simulink model "TVModel_Simulation_21"  (R2021b)
settings: Solver=FixedStepDiscrete  StartTime=0.0  StopTime=250  FixedStep=0.02  MaxStep=0.01  RelTol=1e-3
undefined symbols (not defined in the file or in its folder): MB, TV, TV_OLD
libraries: simulink x22, simulink_extras x14, eeGeneralControl x13, slpidlib x8, fuzblock x4, controlLib x4, cstblocks x3, dspstat3 x2, eeSlidingModeController x1, sharedTrackingLibrary x1
(part 3 of 9)

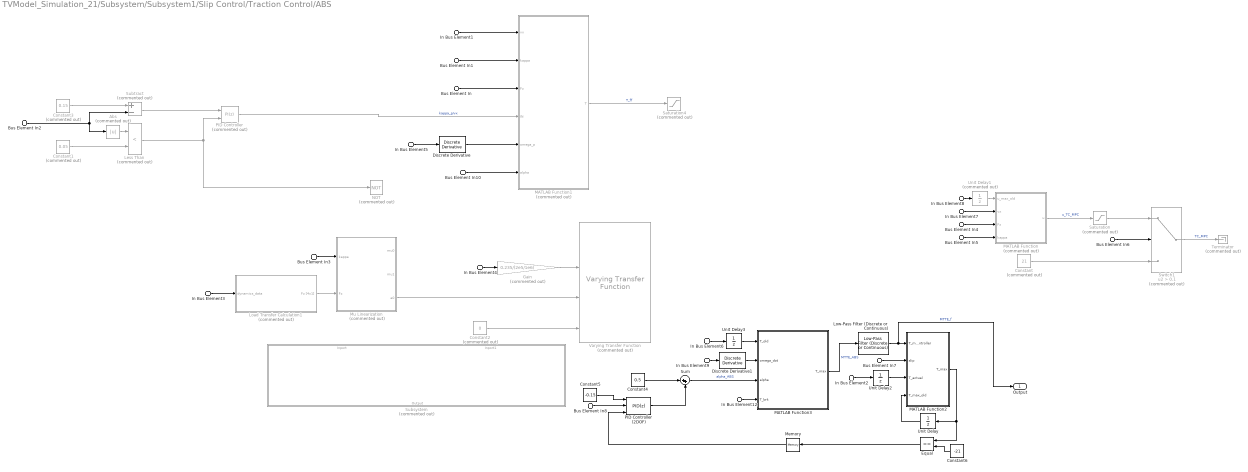
== system TVModel_Simulation_21/Subsystem/Subsystem1/Slip Control/Traction Control/ABS ==
  In Bus Element3 : Inport  PortName=dynamics_data
  In Bus Element1 : Inport  PortName=dynamics_data  Element=vx
  In Bus Element4 : Inport  PortName=dynamics_data  Element=vx
  In Bus Element7 : Inport  PortName=dynamics_data  Element=vx
  In Bus Element5 : Inport  PortName=dynamics_data  Element=omega_wheels
  In Bus Element9 : Inport  PortName=dynamics_data  Element=omega_wheels
  In Bus Element12 : Inport  PortName=dynamics_data  Element=brake_torque
  Bus Element In{1..3,5..8} (7 alike) : Inport  Port=2  PortName=slip_ratio
  Bus Element In10 : Inport  Port=3  PortName=slip_angles
  Bus Element In : Inport  Port=4  PortName=Fz
  Bus Element In4 : Inport  Port=4  PortName=Fz
  In Bus Element8 : Inport  Port=5  PortName=tv
  In Bus Element2 : Inport  Port=5  PortName=tv
  In Bus Element6 : Inport  Port=5  PortName=tv
  Abs : Abs  Commented=on
  Constant : Constant  Commented=on  Value=21
  Constant1 : Constant  Commented=on  Value=0.05
  Constant2 : Constant  Commented=on  Value=0
  Constant3 : Constant  Commented=on  Value=0.15
  Constant4 : Constant  Value=0.5
  Constant5 : Constant  Value=-0.15
  Constant6 : Constant  Value=-21
  Discrete Derivative : simulink/Discrete/Discrete Derivative  gainval=1.0  ICPrevScaledInput=0.0  OutMin=[]  OutMax=[]  OutDataType=fixdt(1, 16)  OutScaling=2^-10  DoSatur=off
  Discrete Derivative1 : simulink/Discrete/Discrete Derivative  gainval=1.0  ICPrevScaledInput=0.0  OutMin=[]  OutMax=[]  OutDataType=fixdt(1, 16)  OutScaling=2^-10  DoSatur=off
  Equal : RelationalOperator  Operator===  OutDataTypeStr=boolean  RndMeth=Simplest
  Gain : Gain  Commented=on  Gain=0.235/(2e5/1e6)
  Less Than : RelationalOperator  Commented=on  Operator=<  OutDataTypeStr=boolean  RndMeth=Simplest
  Load Transfer Calculation1 : Subsystem  Commented=on
  Low-Pass Filter (Discrete or Continuous) : eeGeneralControl/Low-Pass Filter (Discrete or Continuous)  K=1  T=0.1  B=inf  A=-inf  init_option=Inherited from block input  x0=0  Ts=-1
  MATLAB Function : MATLAB Function  Commented=on  TreatAsAtomicUnit=on
  MATLAB Function1 : MATLAB Function  Commented=on  TreatAsAtomicUnit=on
  MATLAB Function2 : MATLAB Function  TreatAsAtomicUnit=on
  MATLAB Function3 : MATLAB Function  TreatAsAtomicUnit=on
  Memory : Memory  InitialCondition=1  InheritSampleTime=on
  Mu Linearization : MATLAB Function  Commented=on  TreatAsAtomicUnit=on
  NOT : Logic  Commented=on  Operator=NOT  IconShape=distinctive  AllPortsSameDT=off  OutDataTypeStr=boolean
  PID Controller : slpidlib/PID Controller  Commented=on  Controller=PI  Form=Parallel  TimeDomain=Discrete-time  UseExternalTs=off  SampleTime=-1  IntegratorMethod=Forward Euler  FilterMethod=Forward Euler  ControllerParametersSource=internal  P=0  I=5  D=0  UseFilter=on  N=100  TunerSelectOption=Transfer Function Based (PID Tuner App)  InitialConditionSource=internal  InitialConditionForIntegrator=0  InitialConditionForFilter=0  DifferentiatorICPrevScaledInput=0  ExternalReset=level  TrackingMode=off  Kt=1  LimitOutput=off  SatLimitsSource=internal  UpperSaturationLimit=0  LowerSaturationLimit=-20  LinearizeAsGain=on  AntiWindupMode=clamping  Kb=1  POutMin=[]  POutMax=[]  IOutMin=[]  IOutMax=[]  DOutMin=[]  DOutMax=[]  NOutMin=[]  NOutMax=[]  SumOutMin=[]  SumOutMax=[]  SaturationOutMin=[]  SaturationOutMax=[]  PParamMin=[]  PParamMax=[]  IParamMin=[]  IParamMax=[]  DParamMin=[]  DParamMax=[]  NParamMin=[]  NParamMax=[]  KbParamMin=[]  KbParamMax=[]  KtParamMin=[]  KtParamMax=[]  KbOutMin=[]  KbOutMax=[]  KtOutMin=[]  KtOutMax=[]  IntegratorOutMin=[]  IntegratorOutMax=[]  FilterOutMin=[]  FilterOutMax=[]  SumI1OutMin=[]  SumI1OutMax=[]  SumI2OutMin=[]  SumI2OutMax=[]  SumI3OutMin=[]  SumI3OutMax=[]  SumI4OutMin=[]  SumI4OutMax=[]  SumDOutMin=[]  SumDOutMax=[]  DifferentiatorOutMin=[]  DifferentiatorOutMax=[]  FilterDiffOutCoefMin=[]  FilterDiffOutCoefMax=[]  ReciprocalOutMin=[]  ReciprocalOutMax=[]  SumDenOutMin=[]  SumDenOutMax=[]  SumNumOutMin=[]  SumNumOutMax=[]  DivideOutMin=[]  DivideOutMax=[]  UdiffTsProdOutMin=[]  UdiffTsProdOutMax=[]  NTsProdOutMin=[]  NTsProdOutMax=[]  UintegralTsProdOutMin=[]  UintegralTsProdOutMax=[]  UngainTsProdOutMin=[]  UngainTsProdOutMax=[]  IntegratorContinuousStateAttributes=''  IntegratorStateMustResolveToSignalObject=off  IntegratorRTWStateStorageClass=Auto  FilterContinuousStateAttributes=''  FilterStateMustResolveToSignalObject=off  FilterRTWStateStorageClass=Auto  ParallelPVariant=InternalParameters  IdealPVariant=Disabled  IVariant=InternalParameters  DVariant=Disabled  IntegratorVariant=Discrete  SatVariant=Disabled  AWVariant=Passthrough  PCopyVariant=Disabled  TRVariant=Disabled  FdbkBlocksVariant=Forward  IdealPFdbkVariant=Disabled  SatFdbkVariant=Disabled  DerivativeFilterVariant=Disabled  NVariant=Disabled  NCopyVariant=Disabled_SignalSpec  FilterICVariant=Disabled  IntegratorICVariant=InternalICs  ExternalResetVariant=ExternalReset  TRSumVariant=Passthrough  SumFdbkVariant=Disabled  SumVariant=Sum_PI  TsampFilterVariant=InternalTs  TsampNgainVariant=Passthrough  TsampIntegralVariant=Passthrough  ExternalSaturationOutDataTypeStr=Inherit: Same as second input
  PID Controller (2DOF) : slpidlib/PID Controller (2DOF)  Controller=PID  Form=Parallel  TimeDomain=Discrete-time  UseExternalTs=off  SampleTime=0.02  IntegratorMethod=Forward Euler  FilterMethod=Forward Euler  ControllerParametersSource=internal  P=1  I=1  D=0  UseFilter=on  N=100  b=1  c=1  TunerSelectOption=Transfer Function Based (PID Tuner App)  InitialConditionSource=internal  InitialConditionForIntegrator=0  InitialConditionForFilter=0  DifferentiatorICPrevScaledInput=0  ExternalReset=level  TrackingMode=off  Kt=1  LimitOutput=on  SatLimitsSource=internal  UpperSaturationLimit=2  LowerSaturationLimit=0  LinearizeAsGain=on  AntiWindupMode=clamping  Kb=1  POutMin=[]  POutMax=[]  IOutMin=[]  IOutMax=[]  DOutMin=[]  DOutMax=[]  NOutMin=[]  NOutMax=[]  bOutMin=[]  bOutMax=[]  cOutMin=[]  cOutMax=[]  SumOutMin=[]  SumOutMax=[]  SaturationOutMin=[]  SaturationOutMax=[]  PParamMin=[]  PParamMax=[]  IParamMin=[]  IParamMax=[]  DParamMin=[]  DParamMax=[]  NParamMin=[]  NParamMax=[]  bParamMin=[]  bParamMax=[]  cParamMin=[]  cParamMax=[]  KbParamMin=[]  KbParamMax=[]  KtParamMin=[]  KtParamMax=[]  KbOutMin=[]  KbOutMax=[]  KtOutMin=[]  KtOutMax=[]  IntegratorOutMin=[]  IntegratorOutMax=[]  FilterOutMin=[]  FilterOutMax=[]  SumI1OutMin=[]  SumI1OutMax=[]  SumI2OutMin=[]  SumI2OutMax=[]  SumI3OutMin=[]  SumI3OutMax=[]  SumI4OutMin=[]  SumI4OutMax=[]  SumDOutMin=[]  SumDOutMax=[]  Sum1OutMin=[]  Sum1OutMax=[]  Sum2OutMin=[]  Sum2OutMax=[]  Sum3OutMin=[]  Sum3OutMax=[]  DifferentiatorOutMin=[]  DifferentiatorOutMax=[]  FilterDiffOutCoefMin=[]  FilterDiffOutCoefMax=[]  ReciprocalOutMin=[]  ReciprocalOutMax=[]  SumDenOutMin=[]  SumDenOutMax=[]  SumNumOutMin=[]  SumNumOutMax=[]  DivideOutMin=[]  DivideOutMax=[]  UdiffTsProdOutMin=[]  UdiffTsProdOutMax=[]  NTsProdOutMin=[]  NTsProdOutMax=[]  UintegralTsProdOutMin=[]  UintegralTsProdOutMax=[]  UngainTsProdOutMin=[]  UngainTsProdOutMax=[]  IntegratorContinuousStateAttributes=''  IntegratorStateMustResolveToSignalObject=off  IntegratorRTWStateStorageClass=Auto  FilterContinuousStateAttributes=''  FilterStateMustResolveToSignalObject=off  FilterRTWStateStorageClass=Auto  ParallelPVariant=InternalParameters  IdealPVariant=Disabled  IVariant=InternalParameters  DVariant=InternalParameters  bVariant=InternalParameters  cVariant=InternalParameters  IntegratorVariant=Discrete  SatVariant=Enabled  AWVariant=DiscClampingParallel  PCopyVariant=Disabled  TRVariant=Disabled  FdbkBlocksVariant=Forward  IdealPFdbkVariant=Disabled  SatFdbkVariant=Disabled  DerivativeFilterVariant=ForwardEulerFilter  NVariant=InternalParameters  NCopyVariant=Disabled  FilterICVariant=InternalICsFilter  IntegratorICVariant=InternalICs  ExternalResetVariant=ExternalReset  TRSumVariant=Passthrough  SumFdbkVariant=Disabled  SumVariant=Sum_PID  TsampFilterVariant=InternalTs  TsampNgainVariant=Passthrough  TsampIntegralVariant=Passthrough  ExternalSaturationOutDataTypeStr=Inherit: Same as second input
      settings: SourceProductBaseCode=SL
  Saturation : Saturate  Commented=on  UpperLimit=21  LowerLimit=0
  Saturation4 : Saturate  Commented=on  UpperLimit=21  LowerLimit=2
  Subsystem : Subsystem  Commented=on
  Subtract : Sum  Commented=on  Inputs=+-
  Sum : Sum  Inputs=|++
  Switch1 : Switch  Commented=on  Criteria=u2 > Threshold  Threshold=0.1
  Terminator : Terminator  Commented=on
  Unit Delay : UnitDelay  SampleTime=-1  HasFrameUpgradeWarning=on
  Unit Delay1 : UnitDelay  Commented=on  SampleTime=-1  HasFrameUpgradeWarning=on
  Unit Delay2 : UnitDelay  SampleTime=-1  HasFrameUpgradeWarning=on
  Unit Delay3 : UnitDelay  SampleTime=-1  HasFrameUpgradeWarning=on
  Varying Transfer Function : cstblocks/Linear Parameter Varying/Varying Transfer Function  Commented=on  N=1
  Output : Outport
  wires:
  Low-Pass Filter (Discrete or Continuous)/1 -> Output/1, MATLAB Function2/1(T_max_controller)  "MTTE_f"
  Constant6/1 -> Equal/2
  Equal/1 -> Memory/1
  Constant5/1 -> PID Controller (2DOF)/1
  Bus Element In8/1 -> PID Controller (2DOF)/2
  Constant4/1 -> Sum/1
  Sum/1 -> MATLAB Function3/3(alpha)  "alpha_ABS"
  Bus Element In4/1 -> MATLAB Function/3(Fz)
  Saturation/1 -> Switch1/1
  Bus Element In6/1 -> Switch1/2
  Constant/1 -> Switch1/3
  MATLAB Function/1(u) -> Saturation/1  "u_TC_MPC"
  Switch1/1 -> Terminator/1  "TC_MPC"
  Unit Delay1/1 -> MATLAB Function/1(u_max_old)
  In Bus Element8/1 -> Unit Delay1/1
  Bus Element In5/1 -> MATLAB Function/4(kappa)
  In Bus Element7/1 -> MATLAB Function/2(vx)
  Less Than/1 -> PID Controller/2, NOT/1
  In Bus Element5/1 -> Discrete Derivative/1
  Mu Linearization/3(a0) -> Varying Transfer Function/3
  Gain/1 -> Varying Transfer Function/2
  In Bus Element4/1 -> Gain/1
  Constant2/1 -> Varying Transfer Function/4
  In Bus Element3/1 -> Load Transfer Calculation1/1(dynamics_data)
  Load Transfer Calculation1/1(Fz [4x1]) -> Mu Linearization/2(Fz)
  Bus Element In3/1 -> Mu Linearization/1(kappa)
  Constant1/1 -> Less Than/2
  Abs/1 -> Less Than/1
  Subtract/1 -> PID Controller/1
  Constant3/1 -> Subtract/1
  Bus Element In2/1 -> Subtract/2, Abs/1
  PID Controller/1 -> MATLAB Function1/4(IN)  "kappa_p/vx"
  Bus Element In10/1 -> MATLAB Function1/6(alpha)
  Bus Element In1/1 -> MATLAB Function1/2(kappa)
  Bus Element In/1 -> MATLAB Function1/3(Fz)
  Discrete Derivative/1 -> MATLAB Function1/5(omega_p)
  In Bus Element1/1 -> MATLAB Function1/1(vx)
  Unit Delay2/1 -> MATLAB Function2/3(T_actual)
  Bus Element In7/1 -> MATLAB Function2/2(slip)
  MATLAB Function1/1(T) -> Saturation4/1  "T_ff"
  In Bus Element2/1 -> Unit Delay2/1
  MATLAB Function2/1(T_max) -> Unit Delay/1, Equal/1
  Unit Delay/1 -> MATLAB Function2/4(T_max_old)
  In Bus Element6/1 -> Unit Delay3/1
  Unit Delay3/1 -> MATLAB Function3/1(T_old)
  In Bus Element9/1 -> Discrete Derivative1/1
  Discrete Derivative1/1 -> MATLAB Function3/2(omega_dot)
  MATLAB Function3/1(T_max) -> Low-Pass Filter (Discrete or Continuous)/1  "MTTE_ABS"
  PID Controller (2DOF)/1 -> Sum/2
  In Bus Element12/1 -> MATLAB Function3/4(T_brk)
  Memory/1 -> PID Controller (2DOF)/3

== system TVModel_Simulation_21/Subsystem/Subsystem1/Slip Control/Traction Control/Fuzzification ==
  kappa_p_FL : Inport
  mu_p_FL : Inport  Port=2
  Fuzzy Logic Controller{,1..3} (4 alike) : fuzblock/Fuzzy Logic  Controller  FIS='TC.fis'  OutputSampleNumber=101  DataType=double  FuzzifiedInputs=off  RuleFiringStrengths=off  RuleOutputs=off  AggregatedOutputs=off  SimulateUsing=Code generation  OutOfRangeInputValueMessage=warning  NoRuleFiredMessage=warning  EmptyOutputFuzzySetMessage=warning
  Mux{,1..3} (4 alike) : Mux  Inputs=2
  Mux4 : Mux
  Selector : Selector  InputPortWidth=4  IndexOptions=Index vector (dialog)  Indices=[1]  OutputSizes=1
  Selector1 : Selector  InputPortWidth=4  IndexOptions=Index vector (dialog)  Indices=[1]  OutputSizes=1
  Selector2 : Selector  InputPortWidth=4  IndexOptions=Index vector (dialog)  Indices=[2]  OutputSizes=1
  Selector3 : Selector  InputPortWidth=4  IndexOptions=Index vector (dialog)  Indices=[2]  OutputSizes=1
  Selector4 : Selector  InputPortWidth=4  IndexOptions=Index vector (dialog)  Indices=[3]  OutputSizes=1
  Selector5 : Selector  InputPortWidth=4  IndexOptions=Index vector (dialog)  Indices=[3]  OutputSizes=1
  Selector6 : Selector  InputPortWidth=4  IndexOptions=Index vector (dialog)  Indices=[4]  OutputSizes=1
  Selector7 : Selector  InputPortWidth=4  IndexOptions=Index vector (dialog)  Indices=[4]  OutputSizes=1
  Unary Minus : UnaryMinus
  kappa_p_FR : InportShadow
  kappa_p_RL : InportShadow
  kappa_p_RR : InportShadow
  mu_p_FR : InportShadow  Port=2
  mu_p_RL : InportShadow  Port=2
  mu_p_RR : InportShadow  Port=2
  Fuzzy_Outputs : Outport
  wires:
  kappa_p_FL/1 -> Selector/1
  Mux/1 -> Fuzzy Logic Controller/1
  mu_p_FL/1 -> Selector1/1
  Fuzzy Logic Controller/1 -> Mux4/1
  Fuzzy Logic Controller1/1 -> Mux4/2
  mu_p_FR/1 -> Selector3/1
  kappa_p_FR/1 -> Selector2/1
  Mux1/1 -> Fuzzy Logic Controller1/1
  Fuzzy Logic Controller2/1 -> Mux4/3
  mu_p_RL/1 -> Selector5/1
  kappa_p_RL/1 -> Selector4/1
  Mux2/1 -> Fuzzy Logic Controller2/1
  Fuzzy Logic Controller3/1 -> Mux4/4
  mu_p_RR/1 -> Selector7/1
  kappa_p_RR/1 -> Selector6/1
  Mux3/1 -> Fuzzy Logic Controller3/1
  Mux4/1 -> Unary Minus/1  "fuzzy_output"
  Selector/1 -> Mux/1
  Selector1/1 -> Mux/2
  Selector2/1 -> Mux1/1
  Selector3/1 -> Mux1/2
  Selector4/1 -> Mux2/1
  Selector5/1 -> Mux2/2
  Selector6/1 -> Mux3/1
  Selector7/1 -> Mux3/2
  Unary Minus/1 -> Fuzzy_Outputs/1

== system TVModel_Simulation_21/Subsystem/Subsystem1/Slip Control/Traction Control/Load Transfer calculation ==
  In Bus Element : Inport  PortName=dynamics_data
  Fz FL : Subsystem
  Fz FR : Subsystem
  Fz RL : Subsystem
  Fz RR : Subsystem
  Mux : Mux
  Fz [4x1] : Outport
  wires:
  Mux/1 -> Fz [4x1]/1
  In Bus Element/1 -> Fz RR/1(dynamics_data), Fz RL/1(dynamics_data), Fz FR/1(dynamics_data), Fz FL/1(dynamics_data)
  Fz FL/1(TV_Info) -> Mux/1  "Fz_FL"
  Fz FR/1(TV_Info) -> Mux/2  "Fz_FR"
  Fz RL/1(TV_Info) -> Mux/3  "Fz_RL"
  Fz RR/1(TV_Info) -> Mux/4  "Fz_RR"

== system TVModel_Simulation_21/Subsystem/Subsystem1/Slip Control/Traction Control/S-R Flip Flops ==
  Set : Inport
  Reset : Inport  Port=2
  Subsystem : Subsystem
  kappa_p : Outport
  wires:
  Set/1 -> Subsystem/1(In1)
  Reset/1 -> Subsystem/2(In2)
  Subsystem/1(Out1) -> kappa_p/1

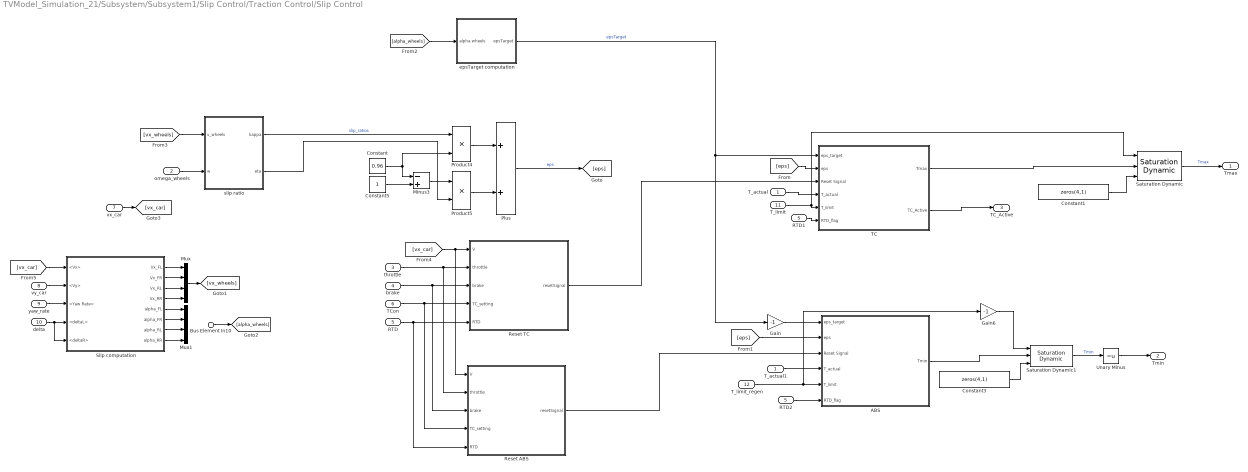
== system TVModel_Simulation_21/Subsystem/Subsystem1/Slip Control/Traction Control/Slip Control ==
  T_actual : Inport  PortDimensions=4
  omega_wheels : Inport  Port=2
  throttle : Inport  Port=3
  brake : Inport  Port=4
  RTD : Inport  Port=5
  TCon : Inport  Port=6
  vx_car : Inport  Port=7
  vy_car : Inport  Port=8
  yaw_rate : Inport  Port=9
  delta : Inport  Port=10
  T_limit : Inport  Port=11
  T_limit_regen : Inport  Port=12
  Bus Element In10 : Inport  Port=13  PortName=slip_angles
  ABS : Subsystem
  Constant : Constant  Value=0.96
  Constant1 : Constant  Value=zeros(4,1)
  Constant3 : Constant  Value=zeros(4,1)
  Constant5 : Constant
  Gain : Gain  Gain=-1
  Gain6 : Gain  Gain=-1
  Minus3 : Sum  Inputs=-+
  Mux : Mux
  Mux1 : Mux
  Plus : Sum
  Product4 : Product
  Product5 : Product
  RTD1 : InportShadow  Port=5
  RTD2 : InportShadow  Port=5
  Reset ABS : Subsystem
  Reset TC : Subsystem
  Saturation Dynamic : simulink/Discontinuities/Saturation Dynamic  OutMin=[]  OutMax=[]  OutDataTypeStr=Inherit: Same as second input  OutDataType=fixdt(1, 16)  OutScaling=2^-10  DoSatur=off
  Saturation Dynamic1 : simulink/Discontinuities/Saturation Dynamic  OutMin=[]  OutMax=[]  OutDataTypeStr=Inherit: Same as second input  OutDataType=fixdt(1, 16)  OutScaling=2^-10  DoSatur=off
  Slip computation : Subsystem
  TC : Subsystem
  T_actual1 : InportShadow  PortDimensions=4
  Unary Minus : UnaryMinus
  epsTarget computation : Subsystem
  slip ratio : Subsystem
  Tmax : Outport
  Tmin : Outport  Port=2
  TC_Active : Outport  Port=3
  wires:
  [eps] -> ABS/2(eps)
  [eps] -> TC/2(eps)
  [alpha_wheels] -> epsTarget computation/1(alpha wheels)
  epsTarget computation/1(epsTarget) -> TC/1(eps_target), Gain/1  "epsTarget"
  T_actual1/1 -> ABS/4(T_actual)
  Minus3/1 -> Product5/1
  Constant5/1 -> Minus3/2
  Reset TC/1(resetSignal) -> TC/3(Reset Signal)
  Constant/1 -> Minus3/1, Product4/2
  Saturation Dynamic/1 -> Tmax/1  "Tmax"
  [vx_car] -> Reset ABS/1(V), Reset TC/1(V)
  [vx_wheels] -> slip ratio/1(v_wheels)
  Reset ABS/1(resetSignal) -> ABS/3(Reset Signal)
  Plus/1 -> [eps]  "eps"
  slip ratio/2(eta) -> Product5/2
  Saturation Dynamic1/1 -> Unary Minus/1  "Tmin"
  Product5/1 -> Plus/2
  brake/1 -> Reset ABS/3(brake), Reset TC/3(brake)
  TCon/1 -> Reset ABS/4(TC_setting), Reset TC/4(TC_setting)
  Product4/1 -> Plus/1
  throttle/1 -> Reset ABS/2(throttle), Reset TC/2(throttle)
  ABS/1(Tmin) -> Saturation Dynamic1/2
  T_actual/1 -> TC/4(T_actual)
  T_limit/1 -> TC/5(T_limit), Saturation Dynamic/1
  omega_wheels/1 -> slip ratio/2(w)
  Constant1/1 -> Saturation Dynamic/3
  RTD/1 -> Reset ABS/5(RTD), Reset TC/5(RTD)
  TC/1(Tmax) -> Saturation Dynamic/2
  Gain/1 -> ABS/1(eps_target)
  T_limit_regen/1 -> ABS/5(T_limit), Gain6/1
  RTD1/1 -> TC/6(RTD_flag)
  RTD2/1 -> ABS/6(RTD_flag)
  Slip computation/1(Vx_FL) -> Mux/1
  Slip computation/2(Vx_FR) -> Mux/2
  Slip computation/3(Vx_RL) -> Mux/3
  Slip computation/4(Vx_RR) -> Mux/4
  Slip computation/5(alpha_FL) -> Mux1/1
  Slip computation/6(alpha_FR) -> Mux1/2
  Slip computation/7(alpha_RL) -> Mux1/3
  Slip computation/8(alpha_RR) -> Mux1/4
  Mux/1 -> [vx_wheels]
  vx_car/1 -> [vx_car]
  [vx_car] -> Slip computation/1(<Vx>)
  vy_car/1 -> Slip computation/2(<Vy>)
  yaw_rate/1 -> Slip computation/3(<Yaw Rate>)
  delta/1 -> Slip computation/5(<deltaR>), Slip computation/4(<deltaL>)
  TC/2(TC_Active) -> TC_Active/1
  Gain6/1 -> Saturation Dynamic1/1
  Constant3/1 -> Saturation Dynamic1/3
  Unary Minus/1 -> Tmin/1
  slip ratio/1(kappa) -> Product4/1  "slip_ratios"
  Bus Element In10/1 -> [alpha_wheels]

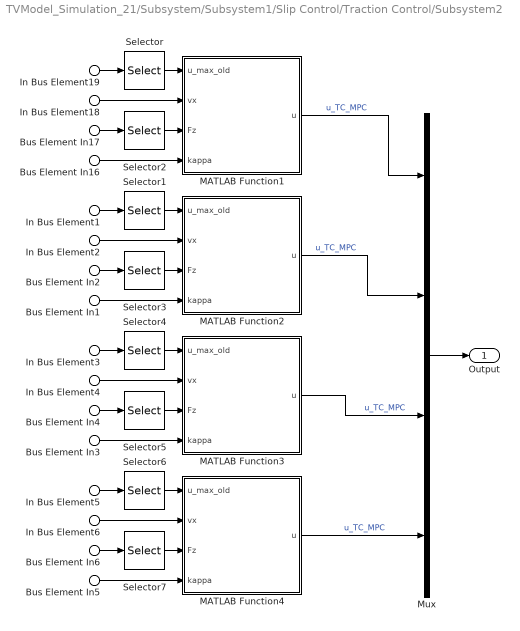
== system TVModel_Simulation_21/Subsystem/Subsystem1/Slip Control/Traction Control/Subsystem2 ==
  In Bus Element{1,3,5,19} (4 alike) : Inport  PortName=tv
  Bus Element In16 : Inport  Port=2  PortName=slip_ratio  Element=fl
  Bus Element In5 : Inport  Port=2  PortName=slip_ratio  Element=rr
  Bus Element In3 : Inport  Port=2  PortName=slip_ratio  Element=rl
  Bus Element In1 : Inport  Port=2  PortName=slip_ratio  Element=fr
  In Bus Element{2,4,6,18} (4 alike) : Inport  Port=3  PortName=dynamics_data  Element=vx
  Bus Element In{2,4,6,17} (4 alike) : Inport  Port=4  PortName=Fz
  MATLAB Function1 : MATLAB Function  TreatAsAtomicUnit=on
  MATLAB Function2 : MATLAB Function  TreatAsAtomicUnit=on
  MATLAB Function3 : MATLAB Function  TreatAsAtomicUnit=on
  MATLAB Function4 : MATLAB Function  TreatAsAtomicUnit=on
  Mux : Mux
  Selector : Selector  InputPortWidth=4  IndexOptions=Index vector (dialog)  Indices=[1]  OutputSizes=1
  Selector1 : Selector  InputPortWidth=4  IndexOptions=Index vector (dialog)  Indices=[2]  OutputSizes=1
  Selector2 : Selector  InputPortWidth=4  IndexOptions=Index vector (dialog)  Indices=[1]  OutputSizes=1
  Selector3 : Selector  InputPortWidth=4  IndexOptions=Index vector (dialog)  Indices=[2]  OutputSizes=1
  Selector4 : Selector  InputPortWidth=4  IndexOptions=Index vector (dialog)  Indices=[3]  OutputSizes=1
  Selector5 : Selector  InputPortWidth=4  IndexOptions=Index vector (dialog)  Indices=[3]  OutputSizes=1
  Selector6 : Selector  InputPortWidth=4  IndexOptions=Index vector (dialog)  Indices=[4]  OutputSizes=1
  Selector7 : Selector  InputPortWidth=4  IndexOptions=Index vector (dialog)  Indices=[4]  OutputSizes=1
  Output : Outport
  wires:
  Mux/1 -> Output/1
  In Bus Element6/1 -> MATLAB Function4/2(vx)
  MATLAB Function4/1(u) -> Mux/4  "u_TC_MPC"
  In Bus Element5/1 -> Selector6/1
  Bus Element In6/1 -> Selector7/1
  Selector6/1 -> MATLAB Function4/1(u_max_old)
  Bus Element In5/1 -> MATLAB Function4/4(kappa)
  Selector7/1 -> MATLAB Function4/3(Fz)
  Selector5/1 -> MATLAB Function3/3(Fz)
  Bus Element In3/1 -> MATLAB Function3/4(kappa)
  Selector4/1 -> MATLAB Function3/1(u_max_old)
  Bus Element In4/1 -> Selector5/1
  In Bus Element3/1 -> Selector4/1
  MATLAB Function3/1(u) -> Mux/3  "u_TC_MPC"
  In Bus Element4/1 -> MATLAB Function3/2(vx)
  In Bus Element2/1 -> MATLAB Function2/2(vx)
  MATLAB Function2/1(u) -> Mux/2  "u_TC_MPC"
  In Bus Element1/1 -> Selector1/1
  Bus Element In2/1 -> Selector3/1
  Selector1/1 -> MATLAB Function2/1(u_max_old)
  Bus Element In1/1 -> MATLAB Function2/4(kappa)
  Selector3/1 -> MATLAB Function2/3(Fz)
  Selector2/1 -> MATLAB Function1/3(Fz)
  Bus Element In16/1 -> MATLAB Function1/4(kappa)
  Selector/1 -> MATLAB Function1/1(u_max_old)
  Bus Element In17/1 -> Selector2/1
  In Bus Element19/1 -> Selector/1
  MATLAB Function1/1(u) -> Mux/1  "u_TC_MPC"
  In Bus Element18/1 -> MATLAB Function1/2(vx)

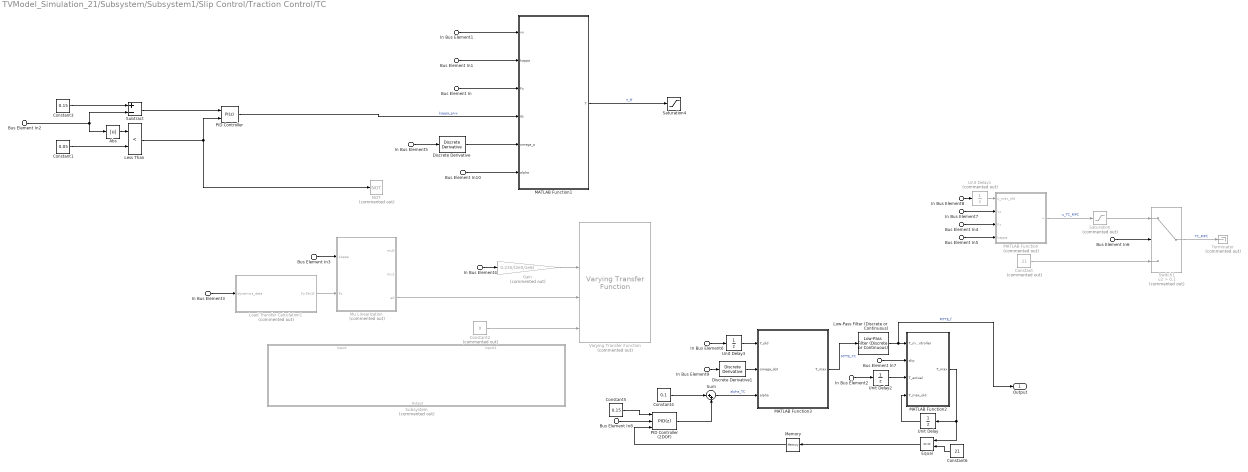
== system TVModel_Simulation_21/Subsystem/Subsystem1/Slip Control/Traction Control/TC ==
  In Bus Element3 : Inport  PortName=dynamics_data
  In Bus Element1 : Inport  PortName=dynamics_data  Element=vx
  In Bus Element4 : Inport  PortName=dynamics_data  Element=vx
  In Bus Element7 : Inport  PortName=dynamics_data  Element=vx
  In Bus Element5 : Inport  PortName=dynamics_data  Element=omega_wheels
  In Bus Element9 : Inport  PortName=dynamics_data  Element=omega_wheels
  Bus Element In{1..3,5..8} (7 alike) : Inport  Port=2  PortName=slip_ratio
  Bus Element In10 : Inport  Port=3  PortName=slip_angles
  Bus Element In : Inport  Port=4  PortName=Fz
  Bus Element In4 : Inport  Port=4  PortName=Fz
  In Bus Element8 : Inport  Port=5  PortName=tv
  In Bus Element2 : Inport  Port=5  PortName=tv
  In Bus Element6 : Inport  Port=5  PortName=tv
  Abs : Abs
  Constant : Constant  Commented=on  Value=21
  Constant1 : Constant  Value=0.05
  Constant2 : Constant  Commented=on  Value=0
  Constant3 : Constant  Value=0.15
  Constant4 : Constant  Value=0.1
  Constant5 : Constant  Value=0.15
  Constant6 : Constant  Value=21
  Discrete Derivative : simulink/Discrete/Discrete Derivative  gainval=1.0  ICPrevScaledInput=0.0  OutMin=[]  OutMax=[]  OutDataType=fixdt(1, 16)  OutScaling=2^-10  DoSatur=off
  Discrete Derivative1 : simulink/Discrete/Discrete Derivative  gainval=1.0  ICPrevScaledInput=0.0  OutMin=[]  OutMax=[]  OutDataType=fixdt(1, 16)  OutScaling=2^-10  DoSatur=off
  Equal : RelationalOperator  Operator===  OutDataTypeStr=boolean  RndMeth=Simplest
  Gain : Gain  Commented=on  Gain=0.235/(2e5/1e6)
  Less Than : RelationalOperator  Operator=<  OutDataTypeStr=boolean  RndMeth=Simplest
  Load Transfer Calculation1 : Subsystem  Commented=on
  Low-Pass Filter (Discrete or Continuous) : eeGeneralControl/Low-Pass Filter (Discrete or Continuous)  K=1  T=0.1  B=inf  A=-inf  init_option=Inherited from block input  x0=0  Ts=-1
  MATLAB Function : MATLAB Function  Commented=on  TreatAsAtomicUnit=on
  MATLAB Function1 : MATLAB Function  TreatAsAtomicUnit=on
  MATLAB Function2 : MATLAB Function  TreatAsAtomicUnit=on
  MATLAB Function3 : MATLAB Function  TreatAsAtomicUnit=on
  Memory : Memory  InitialCondition=1  InheritSampleTime=on
  Mu Linearization : MATLAB Function  Commented=on  TreatAsAtomicUnit=on
  NOT : Logic  Commented=on  Operator=NOT  IconShape=distinctive  AllPortsSameDT=off  OutDataTypeStr=boolean
  PID Controller : slpidlib/PID Controller  Controller=PI  Form=Parallel  TimeDomain=Discrete-time  UseExternalTs=off  SampleTime=-1  IntegratorMethod=Forward Euler  FilterMethod=Forward Euler  ControllerParametersSource=internal  P=0  I=5  D=0  UseFilter=on  N=100  TunerSelectOption=Transfer Function Based (PID Tuner App)  InitialConditionSource=internal  InitialConditionForIntegrator=0  InitialConditionForFilter=0  DifferentiatorICPrevScaledInput=0  ExternalReset=level  TrackingMode=off  Kt=1  LimitOutput=off  SatLimitsSource=internal  UpperSaturationLimit=0  LowerSaturationLimit=-20  LinearizeAsGain=on  AntiWindupMode=clamping  Kb=1  POutMin=[]  POutMax=[]  IOutMin=[]  IOutMax=[]  DOutMin=[]  DOutMax=[]  NOutMin=[]  NOutMax=[]  SumOutMin=[]  SumOutMax=[]  SaturationOutMin=[]  SaturationOutMax=[]  PParamMin=[]  PParamMax=[]  IParamMin=[]  IParamMax=[]  DParamMin=[]  DParamMax=[]  NParamMin=[]  NParamMax=[]  KbParamMin=[]  KbParamMax=[]  KtParamMin=[]  KtParamMax=[]  KbOutMin=[]  KbOutMax=[]  KtOutMin=[]  KtOutMax=[]  IntegratorOutMin=[]  IntegratorOutMax=[]  FilterOutMin=[]  FilterOutMax=[]  SumI1OutMin=[]  SumI1OutMax=[]  SumI2OutMin=[]  SumI2OutMax=[]  SumI3OutMin=[]  SumI3OutMax=[]  SumI4OutMin=[]  SumI4OutMax=[]  SumDOutMin=[]  SumDOutMax=[]  DifferentiatorOutMin=[]  DifferentiatorOutMax=[]  FilterDiffOutCoefMin=[]  FilterDiffOutCoefMax=[]  ReciprocalOutMin=[]  ReciprocalOutMax=[]  SumDenOutMin=[]  SumDenOutMax=[]  SumNumOutMin=[]  SumNumOutMax=[]  DivideOutMin=[]  DivideOutMax=[]  UdiffTsProdOutMin=[]  UdiffTsProdOutMax=[]  NTsProdOutMin=[]  NTsProdOutMax=[]  UintegralTsProdOutMin=[]  UintegralTsProdOutMax=[]  UngainTsProdOutMin=[]  UngainTsProdOutMax=[]  IntegratorContinuousStateAttributes=''  IntegratorStateMustResolveToSignalObject=off  IntegratorRTWStateStorageClass=Auto  FilterContinuousStateAttributes=''  FilterStateMustResolveToSignalObject=off  FilterRTWStateStorageClass=Auto  ParallelPVariant=InternalParameters  IdealPVariant=Disabled  IVariant=InternalParameters  DVariant=Disabled  IntegratorVariant=Discrete  SatVariant=Disabled  AWVariant=Passthrough  PCopyVariant=Disabled  TRVariant=Disabled  FdbkBlocksVariant=Forward  IdealPFdbkVariant=Disabled  SatFdbkVariant=Disabled  DerivativeFilterVariant=Disabled  NVariant=Disabled  NCopyVariant=Disabled_SignalSpec  FilterICVariant=Disabled  IntegratorICVariant=InternalICs  ExternalResetVariant=ExternalReset  TRSumVariant=Passthrough  SumFdbkVariant=Disabled  SumVariant=Sum_PI  TsampFilterVariant=InternalTs  TsampNgainVariant=Passthrough  TsampIntegralVariant=Passthrough  ExternalSaturationOutDataTypeStr=Inherit: Same as second input
  PID Controller (2DOF) : slpidlib/PID Controller (2DOF)  Controller=PID  Form=Parallel  TimeDomain=Discrete-time  UseExternalTs=off  SampleTime=0.02  IntegratorMethod=Forward Euler  FilterMethod=Forward Euler  ControllerParametersSource=internal  P=-2  I=-1  D=0  UseFilter=on  N=100  b=1  c=1  TunerSelectOption=Transfer Function Based (PID Tuner App)  InitialConditionSource=internal  InitialConditionForIntegrator=0  InitialConditionForFilter=0  DifferentiatorICPrevScaledInput=0  ExternalReset=level  TrackingMode=off  Kt=1  LimitOutput=on  SatLimitsSource=internal  UpperSaturationLimit=2  LowerSaturationLimit=0  LinearizeAsGain=on  AntiWindupMode=clamping  Kb=1  POutMin=[]  POutMax=[]  IOutMin=[]  IOutMax=[]  DOutMin=[]  DOutMax=[]  NOutMin=[]  NOutMax=[]  bOutMin=[]  bOutMax=[]  cOutMin=[]  cOutMax=[]  SumOutMin=[]  SumOutMax=[]  SaturationOutMin=[]  SaturationOutMax=[]  PParamMin=[]  PParamMax=[]  IParamMin=[]  IParamMax=[]  DParamMin=[]  DParamMax=[]  NParamMin=[]  NParamMax=[]  bParamMin=[]  bParamMax=[]  cParamMin=[]  cParamMax=[]  KbParamMin=[]  KbParamMax=[]  KtParamMin=[]  KtParamMax=[]  KbOutMin=[]  KbOutMax=[]  KtOutMin=[]  KtOutMax=[]  IntegratorOutMin=[]  IntegratorOutMax=[]  FilterOutMin=[]  FilterOutMax=[]  SumI1OutMin=[]  SumI1OutMax=[]  SumI2OutMin=[]  SumI2OutMax=[]  SumI3OutMin=[]  SumI3OutMax=[]  SumI4OutMin=[]  SumI4OutMax=[]  SumDOutMin=[]  SumDOutMax=[]  Sum1OutMin=[]  Sum1OutMax=[]  Sum2OutMin=[]  Sum2OutMax=[]  Sum3OutMin=[]  Sum3OutMax=[]  DifferentiatorOutMin=[]  DifferentiatorOutMax=[]  FilterDiffOutCoefMin=[]  FilterDiffOutCoefMax=[]  ReciprocalOutMin=[]  ReciprocalOutMax=[]  SumDenOutMin=[]  SumDenOutMax=[]  SumNumOutMin=[]  SumNumOutMax=[]  DivideOutMin=[]  DivideOutMax=[]  UdiffTsProdOutMin=[]  UdiffTsProdOutMax=[]  NTsProdOutMin=[]  NTsProdOutMax=[]  UintegralTsProdOutMin=[]  UintegralTsProdOutMax=[]  UngainTsProdOutMin=[]  UngainTsProdOutMax=[]  IntegratorContinuousStateAttributes=''  IntegratorStateMustResolveToSignalObject=off  IntegratorRTWStateStorageClass=Auto  FilterContinuousStateAttributes=''  FilterStateMustResolveToSignalObject=off  FilterRTWStateStorageClass=Auto  ParallelPVariant=InternalParameters  IdealPVariant=Disabled  IVariant=InternalParameters  DVariant=InternalParameters  bVariant=InternalParameters  cVariant=InternalParameters  IntegratorVariant=Discrete  SatVariant=Enabled  AWVariant=DiscClampingParallel  PCopyVariant=Disabled  TRVariant=Disabled  FdbkBlocksVariant=Forward  IdealPFdbkVariant=Disabled  SatFdbkVariant=Disabled  DerivativeFilterVariant=ForwardEulerFilter  NVariant=InternalParameters  NCopyVariant=Disabled  FilterICVariant=InternalICsFilter  IntegratorICVariant=InternalICs  ExternalResetVariant=ExternalReset  TRSumVariant=Passthrough  SumFdbkVariant=Disabled  SumVariant=Sum_PID  TsampFilterVariant=InternalTs  TsampNgainVariant=Passthrough  TsampIntegralVariant=Passthrough  ExternalSaturationOutDataTypeStr=Inherit: Same as second input
      settings: SourceProductBaseCode=SL
  Saturation : Saturate  Commented=on  UpperLimit=21  LowerLimit=0
  Saturation4 : Saturate  UpperLimit=21  LowerLimit=2
  Subsystem : Subsystem  Commented=on
  Subtract : Sum  Inputs=+-
  Sum : Sum  Inputs=|++
  Switch1 : Switch  Commented=on  Criteria=u2 > Threshold  Threshold=0.1
  Terminator : Terminator  Commented=on
  Unit Delay : UnitDelay  SampleTime=-1  HasFrameUpgradeWarning=on
  Unit Delay1 : UnitDelay  Commented=on  SampleTime=-1  HasFrameUpgradeWarning=on
  Unit Delay2 : UnitDelay  SampleTime=-1  HasFrameUpgradeWarning=on
  Unit Delay3 : UnitDelay  SampleTime=-1  HasFrameUpgradeWarning=on
  Varying Transfer Function : cstblocks/Linear Parameter Varying/Varying Transfer Function  Commented=on  N=1
  Output : Outport
  wires:
  PID Controller (2DOF)/1 -> Sum/2
  MATLAB Function3/1(T_max) -> Low-Pass Filter (Discrete or Continuous)/1  "MTTE_TC"
  Discrete Derivative1/1 -> MATLAB Function3/2(omega_dot)
  In Bus Element9/1 -> Discrete Derivative1/1
  Unit Delay3/1 -> MATLAB Function3/1(T_old)
  In Bus Element6/1 -> Unit Delay3/1
  Unit Delay/1 -> MATLAB Function2/4(T_max_old)
  MATLAB Function2/1(T_max) -> Equal/1, Unit Delay/1
  In Bus Element2/1 -> Unit Delay2/1
  MATLAB Function1/1(T) -> Saturation4/1  "T_ff"
  Bus Element In7/1 -> MATLAB Function2/2(slip)
  Unit Delay2/1 -> MATLAB Function2/3(T_actual)
  In Bus Element1/1 -> MATLAB Function1/1(vx)
  Discrete Derivative/1 -> MATLAB Function1/5(omega_p)
  Bus Element In/1 -> MATLAB Function1/3(Fz)
  Bus Element In1/1 -> MATLAB Function1/2(kappa)
  Bus Element In10/1 -> MATLAB Function1/6(alpha)
  PID Controller/1 -> MATLAB Function1/4(IN)  "kappa_p/vx"
  Bus Element In2/1 -> Abs/1, Subtract/2
  Constant3/1 -> Subtract/1
  Subtract/1 -> PID Controller/1
  Abs/1 -> Less Than/1
  Constant1/1 -> Less Than/2
  Bus Element In3/1 -> Mu Linearization/1(kappa)
  Load Transfer Calculation1/1(Fz [4x1]) -> Mu Linearization/2(Fz)
  In Bus Element3/1 -> Load Transfer Calculation1/1(dynamics_data)
  Constant2/1 -> Varying Transfer Function/4
  In Bus Element4/1 -> Gain/1
  Gain/1 -> Varying Transfer Function/2
  Mu Linearization/3(a0) -> Varying Transfer Function/3
  In Bus Element5/1 -> Discrete Derivative/1
  Less Than/1 -> NOT/1, PID Controller/2
  In Bus Element7/1 -> MATLAB Function/2(vx)
  Bus Element In5/1 -> MATLAB Function/4(kappa)
  In Bus Element8/1 -> Unit Delay1/1
  Unit Delay1/1 -> MATLAB Function/1(u_max_old)
  Switch1/1 -> Terminator/1  "TC_MPC"
  MATLAB Function/1(u) -> Saturation/1  "u_TC_MPC"
  Constant/1 -> Switch1/3
  Bus Element In6/1 -> Switch1/2
  Saturation/1 -> Switch1/1
  Bus Element In4/1 -> MATLAB Function/3(Fz)
  Sum/1 -> MATLAB Function3/3(alpha)  "alpha_TC"
  Constant4/1 -> Sum/1
  Bus Element In8/1 -> PID Controller (2DOF)/2
  Constant5/1 -> PID Controller (2DOF)/1
  Equal/1 -> Memory/1
  Constant6/1 -> Equal/2
  Low-Pass Filter (Discrete or Continuous)/1 -> MATLAB Function2/1(T_max_controller), Output/1  "MTTE_f"
  Memory/1 -> PID Controller (2DOF)/3

== system TVModel_Simulation_21/Subsystem/Subsystem1/Torque Distribution/MPC/     Output Vector Reference ==
  YRD : Inport
  Bus Creator : BusCreator  Inputs=11
  MATLAB Function : MATLAB Function  TreatAsAtomicUnit=on
  VX_ref : Constant  Value=0
  VY_ref : Constant  Value=0
  dT_FL_ref{,1..4} (5 alike) : Constant  Value=0
  dT_FR_ref : Constant  Value=0
  dT_RL_ref : Constant  Value=0
  dT_RR_ref : Constant  Value=0
  y_ref_0 : Outport
  y_ref : Outport  Port=2
  y_ref_e : Outport  Port=3
  Out Bus Element2 : Outport  Port=4  PortName=TV_Info  Element=y_ref
  wires:
  dT_FL_ref4/1 -> Bus Creator/4  "dt_fl_ref"
  dT_FL_ref3/1 -> Bus Creator/5  "dt_fl_ref"
  dT_FL_ref2/1 -> Bus Creator/6  "dt_fl_ref"
  dT_FL_ref1/1 -> Bus Creator/7  "dt_fl_ref"
  dT_RR_ref/1 -> Bus Creator/11
  dT_RL_ref/1 -> Bus Creator/10
  dT_FR_ref/1 -> Bus Creator/9  "dt_fr_ ref"
  dT_FL_ref/1 -> Bus Creator/8
  VX_ref/1 -> Bus Creator/1  "vx_ref"
  VY_ref/1 -> Bus Creator/2  "vy_ref"
  YRD/1 -> Bus Creator/3  "r_ref"
  Bus Creator/1 -> Out Bus Element2/1, y_ref_e/1, MATLAB Function/1(u), y_ref_0/1
  MATLAB Function/1(y) -> y_ref/1

== system TVModel_Simulation_21/Subsystem/Subsystem1/Torque Distribution/MPC/ PRE LUDO ==
  Brake & ESP : Subsystem
  Cross Check1 : MATLAB Function  TreatAsAtomicUnit=on
  Faul Detection : Subsystem
  Hydraulic brakes : Subsystem
  Mz = 0 Bound logic : Subsystem
  Power Calculation Post : Subsystem  Commented=on
  Power Calculation Pre : Subsystem  Commented=on
  Steer_activation : Subsystem  Commented=on

== system TVModel_Simulation_21/Subsystem/Subsystem1/Torque Distribution/MPC/ Parameter Bus  ==
  In Bus Element12 : Inport  PortName=dynamics_data  Element=brake_torque
  In Bus Element7 : Inport  PortName=dynamics_data  Element=omega_wheels
  In Bus Element11 : Inport  Port=2  PortName=front_wheel_angles  Element=single_axis
  In Bus Element25 : Inport  Port=3  PortName=slip_ratio  Element=fl
  In Bus Element1 : Inport  Port=3  PortName=slip_ratio  Element=fr
  In Bus Element2 : Inport  Port=3  PortName=slip_ratio  Element=rl
  In Bus Element3 : Inport  Port=3  PortName=slip_ratio  Element=rr
  Bus Element In1 : Inport  Port=4  PortName=Fz
  Bus p : Subsystem
  Constant : Constant  Value=0.8
  Demux : Demux
  Demux1 : Demux
  Demux2 : Demux
  Gain : Gain  Gain=13.5
  Mux : Mux  Inputs=TV.MPC.np
  Signal Specification{4..7} (4 alike) : SignalSpecification  Dimensions=1
  p : Outport
  Out Bus Element6 : Outport  Port=2  PortName=TV_Info  Element=p
  wires:
  In Bus Element11/1 -> Mux/1  "wheel_angle_single_axis"
  Bus p/1(TV_Info) -> Out Bus Element6/1, p/1
  Demux/1 -> Signal Specification4/1
  Demux/2 -> Signal Specification5/1
  Demux/3 -> Signal Specification6/1
  Demux/4 -> Signal Specification7/1
  Signal Specification4/1 -> Mux/6  "brake_torque_fl"
  Signal Specification5/1 -> Mux/7  "brake_torque_fr"
  Signal Specification6/1 -> Mux/8  "brake_torque_rl"
  Signal Specification7/1 -> Mux/9  "brake_torque_rr"
  Mux/1 -> Bus p/1(In)
  In Bus Element12/1 -> Demux/1
  In Bus Element7/1 -> Gain/1
  Gain/1 -> Demux1/1
  In Bus Element25/1 -> Mux/2
  In Bus Element1/1 -> Mux/3
  In Bus Element2/1 -> Mux/4
  In Bus Element3/1 -> Mux/5
  Constant/1 -> Mux/18
  Demux2/4 -> Mux/13
  Demux2/3 -> Mux/12
  Demux2/2 -> Mux/11
  Demux2/1 -> Mux/10
  Bus Element In1/1 -> Demux2/1
  Demux1/1 -> Mux/14  "slip_ratio_fl"
  Demux1/2 -> Mux/15  "slip_ratio_fr"
  Demux1/3 -> Mux/16  "slip_ratio_rl"
  Demux1/4 -> Mux/17  "slip_ratio_rr"

== system TVModel_Simulation_21/Subsystem/Subsystem1/Torque Distribution/MPC/ States ==
  motor_torque : Inport
  In Bus Element26 : Inport  Port=2  PortName=dynamics_data  Element=vx
  In Bus Element1 : Inport  Port=2  PortName=dynamics_data  Element=vy
  In Bus Element2 : Inport  Port=2  PortName=dynamics_data  Element=yaw_rate
  Bus Creator1 : BusCreator  Inputs=7
  Demux : Demux
  Saturation : Saturate  UpperLimit=inf  LowerLimit=2
  x : Outport
  Out Bus Element6 : Outport  Port=2  PortName=TV_Info  Element=x
  wires:
  Saturation/1 -> Bus Creator1/1
  In Bus Element26/1 -> Saturation/1
  In Bus Element2/1 -> Bus Creator1/3
  In Bus Element1/1 -> Bus Creator1/2
  Bus Creator1/1 -> Out Bus Element6/1, x/1
  motor_torque/1 -> Demux/1
  Demux/4 -> Bus Creator1/7  "t_rr"
  Demux/3 -> Bus Creator1/6  "t_rl"
  Demux/2 -> Bus Creator1/5  "t_fr"
  Demux/1 -> Bus Creator1/4  "t_fl"

== system TVModel_Simulation_21/Subsystem/Subsystem1/Torque Distribution/MPC/Control Constraints ==
  Constant : Constant  Value=100000*ones(4,1)
  Constant1 : Constant  Value=TV.MPC.N
  MATLAB Function1 : MATLAB Function  TreatAsAtomicUnit=on
  Unary Minus : UnaryMinus
  lbu : Outport
  ubu : Outport  Port=2
  Out Bus Element19 : Outport  Port=3  PortName=TV_Info  Element=lbu
  Out Bus Element1 : Outport  Port=3  PortName=TV_Info  Element=ubu
  wires:
  Unary Minus/1 -> Out Bus Element19/1, lbu/1
  Constant/1 -> MATLAB Function1/1(u)
  MATLAB Function1/1(y) -> Unary Minus/1, Out Bus Element1/1, ubu/1
  Constant1/1 -> MATLAB Function1/2(N)

== system TVModel_Simulation_21/Subsystem/Subsystem1/Torque Distribution/MPC/Faults Detection ==
  OCP Status : Inport
  In Bus throttle : Inport  Port=2  PortName=driver_inputs
  In Bus Element1 : Inport  Port=2  PortName=driver_inputs  Element=throttle
  In Bus Element4 : Inport  Port=2  PortName=driver_inputs  Element=brake
  In Bus Element2 : Inport  Port=3  PortName=dynamics_data
  In Bus Element7 : Inport  Port=3  PortName=dynamics_data
  In Bus Element6 : Inport  Port=4  PortName=brake_signal
  In Bus Element9 : Inport  Port=5  PortName=hv
  In Bus torque_map3 : Inport  Port=6  PortName=car_settings
  X1 : Inport  Port=7
  Bus Element In : Inport  Port=8  PortName=Tire_Bounds
  Constant : Constant
  Constant1 : Constant  Value=0.05
  Divide : Product  Inputs=**
  If : If  IfExpression=u1 == 1  ElseIfExpressions=u1 == 2  ShowElse=off
  Less Than3 : RelationalOperator  Operator=>  OutDataTypeStr=boolean  RndMeth=Simplest
  MPC : Subsystem  TreatAsAtomicUnit=on
  Merge : Merge
  Overlap Chart : Stateflow chart  TreatAsAtomicUnit=on
  Selector : Selector  InputPortWidth=7  IndexOptions=Index vector (dialog)  Indices=[4:7]  OutputSizes=1
  Simple torque : Subsystem  TreatAsAtomicUnit=on
  Subsystem : Subsystem
  Torque : Outport
  Out Bus Element8 : Outport  Port=2  PortName=TV_Info  Element=torque_flag
  wires:
  Bus Element In/1 -> Simple torque/6(Tire_Bounds)
  Constant/1 -> Divide/2
  In Bus Element1/1 -> Overlap Chart/1(throttle)  "throttle_pre"
  In Bus Element4/1 -> Less Than3/1
  Divide/1 -> Torque/1
  Overlap Chart/1(torque_flag) -> Out Bus Element8/1
  Less Than3/1 -> Overlap Chart/2(brake)
  Constant1/1 -> Less Than3/2
  X1/1 -> Selector/1  "Torque"
  Subsystem/1(TV Mode Selection) -> If/1  "Mode_Selector"
  If/2 -> Simple torque/Action
  If/1 -> MPC/Action
  OCP Status/1 -> Subsystem/1(OCP Status)
  Simple torque/1(Out1) -> Merge/2
  MPC/1(Out1) -> Merge/1
  Merge/1 -> Divide/1
  In Bus throttle/1 -> Simple torque/1(driver_inputs)
  In Bus Element2/1 -> Simple torque/2(dynamics_data)
  In Bus Element9/1 -> Simple torque/4(hv)
  In Bus Element6/1 -> Simple torque/3(brake_signal)
  In Bus torque_map3/1 -> Simple torque/5(car_settings)
  In Bus Element7/1 -> Subsystem/2(dynamics_data)
  Selector/1 -> MPC/1(X1)

== system TVModel_Simulation_21/Subsystem/Subsystem1/Torque Distribution/MPC/Mz Generation ==
  In Bus Element2 : Inport  PortName=dynamics_data
  In Bus Element8 : Inport  Port=2  PortName=front_wheel_angles  Element=single_axis
  In Bus Element14 : Inport  Port=2  PortName=front_wheel_angles  Element=different_axis
  In Bus Element13 : Inport  Port=2  PortName=front_wheel_angles  Element=different_axis
  Bus Element In3 : Inport  Port=3  PortName=Torque_Bounds  Element=lbx
  Bus Element In1 : Inport  Port=3  PortName=Torque_Bounds  Element=lbx
  Bus Element In2 : Inport  Port=3  PortName=Torque_Bounds  Element=ubx
  Bus Element In4 : Inport  Port=3  PortName=Torque_Bounds  Element=ubx
  Constant2 : Constant  Value=50
  MATLAB Function : MATLAB Function  TreatAsAtomicUnit=on
  MATLAB Function3 : MATLAB Function  TreatAsAtomicUnit=on
  MATLAB Function4 : MATLAB Function  TreatAsAtomicUnit=on
  Product1 : Product
  Saturation Dynamic : simulink/Discontinuities/Saturation Dynamic  OutMin=[]  OutMax=[]  OutDataTypeStr=Inherit: Same as second input  OutDataType=fixdt(1, 16)  OutScaling=2^-10  DoSatur=off
  Steer Activation : Subsystem
  Out Bus Element : Outport  PortName=mz  Element=lb
  Out Bus Element1 : Outport  PortName=mz  Element=ub
  Out Bus Element4 : Outport  Port=2  PortName=TV_Info  Element=mz_ub
  Out Bus Element5 : Outport  Port=2  PortName=TV_Info  Element=mz_lb
  Out Bus Element6 : Outport  Port=3  PortName=epsilon
  wires:
  Saturation Dynamic/1 -> MATLAB Function/1(u)  "Mz_lim"
  MATLAB Function3/1(Mzlim) -> Saturation Dynamic/3  "Mz_LIM_lower"
  Product1/1 -> Saturation Dynamic/2  "mz_output"
  Bus Element In1/1 -> MATLAB Function3/2(lbx)
  In Bus Element14/1 -> MATLAB Function4/3(delta)
  MATLAB Function4/1(Mzlim) -> Saturation Dynamic/1  "Mz_LIM_upper"
  Bus Element In3/1 -> MATLAB Function4/2(lbx)
  In Bus Element13/1 -> MATLAB Function3/3(delta)
  Bus Element In4/1 -> MATLAB Function3/1(ubx)
  Bus Element In2/1 -> MATLAB Function4/1(ubx)
  Constant2/1 -> Product1/1
  In Bus Element2/1 -> Steer Activation/2(dynamics_data)
  Steer Activation/1(epsilon) -> Out Bus Element6/1, Product1/2, MATLAB Function/2(epsilon)  "epsilon"
  In Bus Element8/1 -> Steer Activation/1(front_wheel_angle)
  MATLAB Function/1(Mzlb) -> Out Bus Element/1, Out Bus Element5/1
  MATLAB Function/2(Mzub) -> Out Bus Element4/1, Out Bus Element1/1

== system TVModel_Simulation_21/Subsystem/Subsystem1/Torque Distribution/MPC/Nonlinear constraints_0 ==
  Constant : Constant  Value=[1e4;8e5;1e4;1e4;1e4;0.1]
  Unary Minus : UnaryMinus
  lh_0 : Outport
  uh_0 : Outport  Port=2
  wires:
  Unary Minus/1 -> lh_0/1
  Constant/1 -> uh_0/1, Unary Minus/1

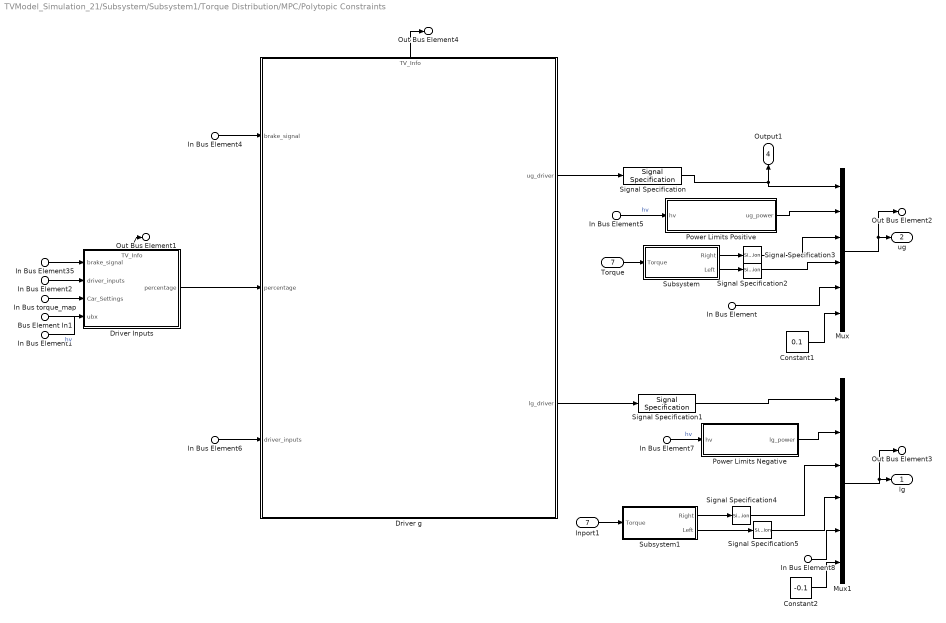
== system TVModel_Simulation_21/Subsystem/Subsystem1/Torque Distribution/MPC/Polytopic Constraints ==
  In Bus Element5 : Inport  PortName=hv
  In Bus Element7 : Inport  PortName=hv
  In Bus Element1 : Inport  PortName=hv
  In Bus Element35 : Inport  Port=2  PortName=brake_signal
  In Bus Element4 : Inport  Port=2  PortName=brake_signal
  In Bus Element2 : Inport  Port=3  PortName=driver_inputs
  In Bus Element6 : Inport  Port=3  PortName=driver_inputs
  In Bus torque_map : Inport  Port=4  PortName=Car_Settings
  In Bus Element : Inport  Port=5  PortName=mz  Element=ub
  In Bus Element8 : Inport  Port=5  PortName=mz  Element=lb
  Bus Element In1 : Inport  Port=6  PortName=T_max
  Torque : Inport  Port=7
  Constant1 : Constant  Value=0.1
  Constant2 : Constant  Value=-0.1
  Driver Inputs : Subsystem
      settings: PortSchema="{\"entries\":[{\"content\":{\"sides\":[{\"content\":{\"connectorIds\":[\"In1\",\"In2\",\"In3\",\"In4\"]},\"type\":\"ConnectorPlacement.EquallySpacedRectSide\",\"uuid\":\"334783ee-11f3-4144-8a14-28dc56086a4b\"},{\"content\":{\"connectorIds\":[\"Out1\"],\"side\":\"RIGHT\"},\"type\":\"ConnectorPlacement.EquallySpacedRectSide\",\"uuid\":\"49c8e620-bd09-4fee-a8d6-6c7a5f6563c1\"},{\"content\":{\"connectorIds\":[\"Out2\"],\"side\":\"TOP\"},\"type\":\"ConnectorPlacement.EquallySpacedRectSide\",\"uuid\":\"cef52ef8-f6f7-4321-a9c9-502de0ffc851\"}]},\"type\":\"ConnectorPlacement.EquallySpacedConnector\",\"uuid\":\"45428ca6-b9a3-4f64-8f7b-2072997d615d\"}],\"packageUris\":[\"http://schema.mathworks.com/mf0/Connector/R2020b\"],\"version\":\"1.0\"}"
  Driver g : Subsystem
      settings: PortSchema="{\"entries\":[{\"content\":{\"sides\":[{\"content\":{\"connectorIds\":[\"In1\",\"In2\",\"In3\"]},\"type\":\"ConnectorPlacement.EquallySpacedRectSide\",\"uuid\":\"52593113-81e3-4b2d-919c-0421b1274de7\"},{\"content\":{\"connectorIds\":[\"Out1\",\"Out2\"],\"side\":\"RIGHT\"},\"type\":\"ConnectorPlacement.EquallySpacedRectSide\",\"uuid\":\"003691be-7065-493d-8a97-6bcaaf8c0f8d\"},{\"content\":{\"connectorIds\":[\"Out3\"],\"side\":\"TOP\"},\"type\":\"ConnectorPlacement.EquallySpacedRectSide\",\"uuid\":\"77e10d31-2af4-42f4-ba5d-4e60bb02d914\"}]},\"type\":\"ConnectorPlacement.EquallySpacedConnector\",\"uuid\":\"ad322a89-c7fc-4aff-bfd3-29198c6c5477\"}],\"packageUris\":[\"http://schema.mathworks.com/mf0/Connector/R2020b\"],\"version\":\"1.0\"}"
  Inport1 : InportShadow  Port=7
  Mux : Mux  Inputs=6
  Mux1 : Mux  Inputs=6
  Power Limits Negative : Subsystem
  Power Limits Positive : Subsystem
  Signal Specification{,1..5} (6 alike) : SignalSpecification  Dimensions=1
  Subsystem : Subsystem
  Subsystem1 : Subsystem
  lg : Outport
  ug : Outport  Port=2
  Out Bus Element1 : Outport  Port=3  PortName=TV_Info  Element=Driver_Inputs
  Out Bus Element2 : Outport  Port=3  PortName=TV_Info  Element=ug
  Out Bus Element3 : Outport  Port=3  PortName=TV_Info  Element=lg
  Out Bus Element4 : Outport  Port=3  PortName=TV_Info  Element=Driver_g
  Output1 : Outport  Port=4
  wires:
  In Bus Element8/1 -> Mux1/5
  Signal Specification5/1 -> Mux1/4
  Signal Specification4/1 -> Mux1/3
  Signal Specification1/1 -> Mux1/1
  In Bus Element/1 -> Mux/5
  Signal Specification2/1 -> Mux/4
  Signal Specification3/1 -> Mux/3
  Driver Inputs/1(percentage) -> Driver g/2(percentage)
  Inport1/1 -> Subsystem1/1(Torque)
  Torque/1 -> Subsystem/1(Torque)
  Driver g/2(lg_driver) -> Signal Specification1/1
  Driver g/1(ug_driver) -> Signal Specification/1
  Mux/1 -> Out Bus Element2/1, ug/1
  Mux1/1 -> lg/1, Out Bus Element3/1
  In Bus Element35/1 -> Driver Inputs/1(brake_signal)
  In Bus Element2/1 -> Driver Inputs/2(driver_inputs)
  In Bus torque_map/1 -> Driver Inputs/3(Car_Settings)
  In Bus Element4/1 -> Driver g/1(brake_signal)
  In Bus Element6/1 -> Driver g/3(driver_inputs)
  Driver Inputs/2(TV_Info) -> Out Bus Element1/1
  Driver g/3(TV_Info) -> Out Bus Element4/1
  Bus Element In1/1 -> Driver Inputs/4(ubx)
  Subsystem/2(Left) -> Signal Specification2/1
  Subsystem/1(Right) -> Signal Specification3/1
  Subsystem1/1(Right) -> Signal Specification4/1
  Subsystem1/2(Left) -> Signal Specification5/1
  In Bus Element1/1 -> ?  "hv"
  Signal Specification/1 -> Mux/1, Output1/1
  Power Limits Negative/1(lg_power) -> Mux1/2
  In Bus Element7/1 -> Power Limits Negative/1(hv)  "hv"
  Power Limits Positive/1(ug_power) -> Mux/2
  In Bus Element5/1 -> Power Limits Positive/1(hv)  "hv"
  Constant1/1 -> Mux/6
  Constant2/1 -> Mux1/6

== system TVModel_Simulation_21/Subsystem/Subsystem1/Torque Distribution/MPC/Slack variables Weights  ==
  Constant : Constant  Value=[1;5;5;1e-3]
  zl_e : Outport
  zu_e : Outport  Port=2
  wires:
  Constant/1 -> zl_e/1, zu_e/1
